simulink model "Model_StateSpace"  (R2019a)
settings: Solver=FixedStepAuto  StartTime=0.0  StopTime=10  FixedStep=0.01  RelTol=1e-3
undefined symbols (not defined in the file or in its folder): A1, B1, C1
settings Model: Creator=Tyson  LastModifiedBy=Tyson

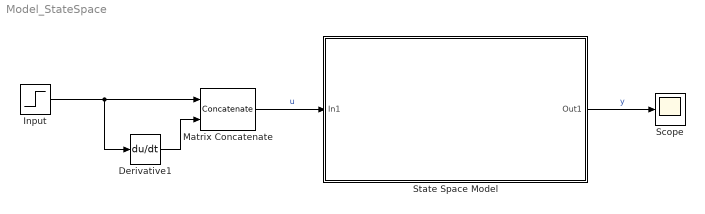
== system Model_StateSpace ==
  Derivative1 : Derivative
  Input : Step  After=5  SampleTime=0
  Matrix Concatenate : Concatenate  Mode=Multidimensional array  ConcatenateDimension=2
  Scope : Scope
  State Space Model : Subsystem
  wires:
  Derivative1/1 -> Matrix Concatenate/2
  Input/1 -> Matrix Concatenate/1, Derivative1/1
  Matrix Concatenate/1 -> State Space Model/1(In1)  "u"
  State Space Model/1(Out1) -> Scope/1  "y"

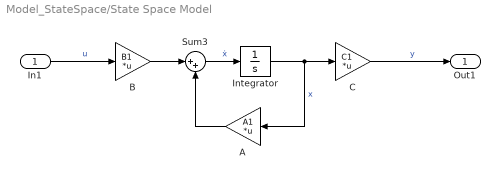
== system Model_StateSpace/State Space Model ==
  In1 : Inport
  A : Gain  Gain=A1  Multiplication=Matrix(K*u)
  B : Gain  Gain=B1  Multiplication=Matrix(K*u)
  C : Gain  Gain=C1  Multiplication=Matrix(K*u)
  Integrator : Integrator
  Sum3 : Sum  Inputs=|++
  Out1 : Outport
  wires:
  In1/1 -> B/1  "u"
  B/1 -> Sum3/1
  A/1 -> Sum3/2
  Sum3/1 -> Integrator/1  "ẋ"
  C/1 -> Out1/1  "y"
  Integrator/1 -> C/1, A/1  "x"
